simulink model "PitchHarness"  (R2023a)
settings: Solver=ode4  StartTime=0.0  StopTime=100  FixedStep=dt  RelTol=1e-3
undefined symbols (not defined in the file): Pitch, TO
libraries: Actuators x1, PitchController x1, simulink_extras x1, Telemaster_Lib x1
settings Model: Creator=igmso  LastModifiedBy=igmso
settings DataIOCC: ExternalInput=[t,u]  InitialState=getstatestruct(SteadyState(idx).op)  SaveFormat=StructureWithTime

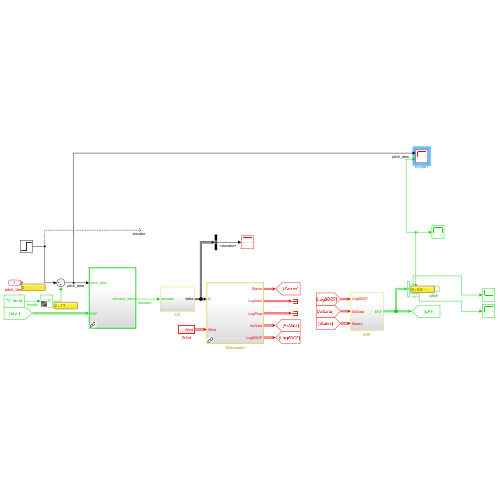
[thumbnail: Simulink's stored preview of the top-level diagram]
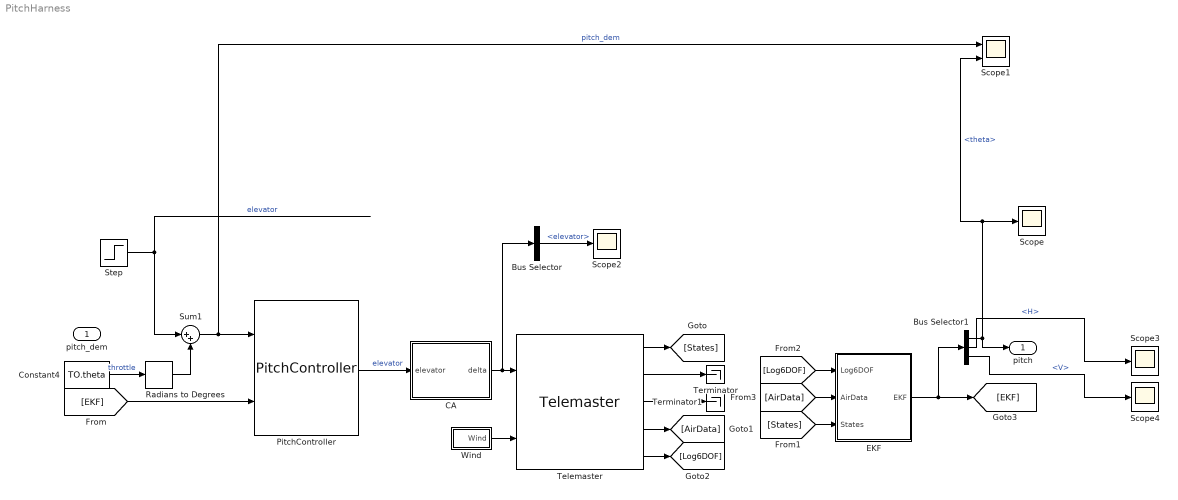
== system PitchHarness ==
  pitch_dem : Inport
  Bus Selector : BusSelector  OutputSignals=elevator
  Bus Selector1 : BusSelector  OutputSignals=States.theta,H,V
  CA : Subsystem  SystemSampleTime=1/400
  Constant4 : Constant  Value=TO.theta  SampleTime=1/400
  EKF : Subsystem
  PitchController : PitchController/PitchController  SystemSampleTime=1/Pitch.ControlRate  VariantActivationTime=update diagram  Latency=0  AutoFrameSizeCalculation=off
  Radians to Degrees : simulink_extras/Transformations/Radians to Degrees
  Scope{,2..4} (4 alike) : Scope
  Scope1 : Scope  NumInputPorts=2
  Step : Step  After=15  SampleTime=0
  Sum1 : Sum  Inputs=|++
  Telemaster : Telemaster_Lib/Telemaster  SystemSampleTime=-1  VariantActivationTime=update diagram  Latency=0  AutoFrameSizeCalculation=off
  Terminator : Terminator
  Terminator1 : Terminator
  Wind : Subsystem  TreatAsAtomicUnit=on  SystemSampleTime=1/4000
  pitch : Outport
  wires:
  Telemaster/3 -> Terminator1/1
  [States] -> EKF/3(States)
  Telemaster/2 -> Terminator/1
  [AirData] -> EKF/2(AirData)
  Telemaster/1 -> [States]
  [Log6DOF] -> EKF/1(Log6DOF)
  Telemaster/5 -> [Log6DOF]
  Telemaster/4 -> [AirData]
  Step/1 -> Sum1/1  "elevator"
  [EKF] -> PitchController/2
  Sum1/1 -> Scope1/1, PitchController/1  "pitch_dem"
  Wind/1(Wind) -> Telemaster/2
  EKF/1(EKF) -> Bus Selector1/1, [EKF]
  Bus Selector1/1 -> pitch/1, Scope1/2, Scope/1  "<theta>"
  Constant4/1 -> Radians to Degrees/1  "throttle"
  Radians to Degrees/1 -> Sum1/2
  CA/1(delta) -> Bus Selector/1, Telemaster/1
  Bus Selector/1 -> Scope2/1  "<elevator>"
  Bus Selector1/2 -> Scope3/1  "<H>"
  Bus Selector1/3 -> Scope4/1  "<V>"
  PitchController/1 -> CA/1(elevator)  "elevator"

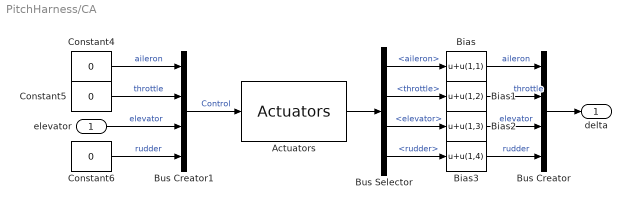
== system PitchHarness/CA ==
  elevator : Inport
  Actuators : Actuators/Actuators  SystemSampleTime=-1  VariantActivationTime=update diagram  Latency=0  AutoFrameSizeCalculation=off
  Bias : Bias  Bias=u(1,1)  SaturateOnIntegerOverflow=off
  Bias1 : Bias  Bias=u(1,2)  SaturateOnIntegerOverflow=off
  Bias2 : Bias  Bias=u(1,3)  SaturateOnIntegerOverflow=off
  Bias3 : Bias  Bias=u(1,4)  SaturateOnIntegerOverflow=off
  Bus Selector : BusSelector  OutputSignals=aileron,throttle,elevator,rudder
  Bus Creator : BusCreator  Inputs=4
  Bus Creator1 : BusCreator  Inputs=4
  Constant4 : Constant  Value=0  SampleTime=1/400
  Constant5 : Constant  Value=0  SampleTime=1/400
  Constant6 : Constant  Value=0  SampleTime=1/400
  delta : Outport
  wires:
  Constant6/1 -> Bus Creator1/4  "rudder"
  Constant4/1 -> Bus Creator1/1  "aileron"
  elevator/1 -> Bus Creator1/3  "elevator"
  Bus Creator1/1 -> Actuators/1  "Control"
  Constant5/1 -> Bus Creator1/2  "throttle"
  Actuators/1 -> Bus Selector/1
  Bus Selector/1 -> Bias/1  "<aileron>"
  Bus Selector/2 -> Bias1/1  "<throttle>"
  Bus Selector/3 -> Bias2/1  "<elevator>"
  Bus Selector/4 -> Bias3/1  "<rudder>"
  Bias/1 -> Bus Creator/1  "aileron"
  Bias1/1 -> Bus Creator/2  "throttle"
  Bias2/1 -> Bus Creator/3  "elevator"
  Bias3/1 -> Bus Creator/4  "rudder"
  Bus Creator/1 -> delta/1

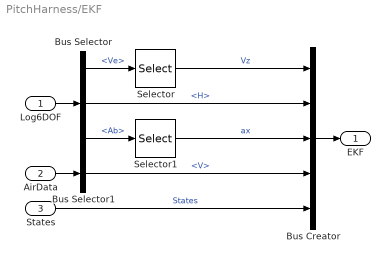
== system PitchHarness/EKF ==
  Log6DOF : Inport
  AirData : Inport  Port=2
  States : Inport  Port=3
  Bus Selector : BusSelector  OutputSignals=Ve,H,Ab
  Bus Selector1 : BusSelector  OutputSignals=V
  Bus Creator : BusCreator  Inputs=5
  Selector : Selector  InputPortWidth=3  IndexOptions=Index vector (dialog)  Indices=3  OutputSizes=1
  Selector1 : Selector  InputPortWidth=3  IndexOptions=Index vector (dialog)  Indices=1  OutputSizes=1
  EKF : Outport  SampleTime=1/400
  wires:
  Bus Selector/1 -> Selector/1  "<Ve>"
  Selector1/1 -> Bus Creator/3  "ax"
  Bus Selector/3 -> Selector1/1  "<Ab>"
  Log6DOF/1 -> Bus Selector/1
  Bus Selector1/1 -> Bus Creator/4  "<V>"
  Bus Selector/2 -> Bus Creator/2  "<H>"
  AirData/1 -> Bus Selector1/1
  Bus Creator/1 -> EKF/1
  Selector/1 -> Bus Creator/1  "Vz"
  States/1 -> Bus Creator/5  "States"

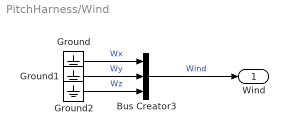
== system PitchHarness/Wind ==
  Bus Creator3 : BusCreator  Inputs=3
  Ground : Ground
  Ground1 : Ground
  Ground2 : Ground
  Wind : Outport
  wires:
  Ground1/1 -> Bus Creator3/2  "Wy"
  Ground2/1 -> Bus Creator3/3  "Wz"
  Bus Creator3/1 -> Wind/1  "Wind"
  Ground/1 -> Bus Creator3/1  "Wx"
